simulink model "RefModel_AeroDyn_Sim"  (R2020b)
settings: Solver=ode1  StartTime=tspan(1)  StopTime=inf  FixedStep=1/sensorFs.imuUpdateFs  RelTol=1e-3  EnableMultiTasking=on
undefined symbols (not defined in the file or in its folder): ACTUATOR_SET, Earth, ENVIRONMENT_SET, F, Light, MIL, sensorFs, SIM_SENSOR_SET, UAVPARAM_SET, WGS84
libraries: simulink x10, aerolibactuator x9, aerolibnav x6, sharedutil x5, shared6dofsys x3, aerolibwind2 x2, aerolibasang x2, aerolibatmos2 x1, aerolibconvert2 x1, aerolibgravity2 x1, aerolibtransform2 x1
(part 1 of 3)
settings Model: PauseTimes=[10 20]  Creator=sl  LastModifiedBy=sl
settings SolverCC: AutoInsertRateTranBlk=on
settings OptimizationCC: DefaultParameterBehavior=Inlined  EnhancedBackFolding=on  PassReuseOutputArgsAs=Individual arguments  ZeroExternalMemoryAtStartup=off  ZeroInternalMemoryAtStartup=off  MaxStackSize=64  OptimizeBlockOrder=speed  DifferentSizesBufferReuse=on  EfficientTunableParamExpr=on
settings DebuggingCC: MultiTaskCondExecSysMsg=none  ParameterTunabilityLossMsg=error  UnconnectedInputMsg=none  UnconnectedOutputMsg=none  UnconnectedLineMsg=none
settings HardwareCC: ProdBitPerPointer=32  ProdBitPerSizeT=32  ProdBitPerPtrDiffT=32  ProdLargestAtomicInteger=Long  ProdLargestAtomicFloat=Double  ProdWordSize=32  ProdHWDeviceType=ARM Compatible->ARM Cortex
settings SFSimCC: MATLABDynamicMemAlloc=off
settings RTWCC: Description=Embedded Coder  SystemTargetFile=ert.tlc  TemplateMakefile=ert_default_tmf  GenerateReport=on  Toolchain=GNU Tools for ARM Embedded Processors  IncludeHyperlinkInReport=on  LaunchReport=on  GenerateTraceInfo=on  GenerateTraceReport=on  GenerateTraceReportSl=on  GenerateTraceReportSf=on  GenerateTraceReportEml=on
settings CodeAppCC: ForceParamTrailComments=on  IgnoreCustomStorageClasses=off  OperatorAnnotations=on  SimulinkDataObjDesc=on  SFDataObjDesc=on  InsertBlockDesc=on
settings ERTTargetCC: InlinedParameterPlacement=NonHierarchical  ERTCustomFileTemplate=example_file_process.tlc

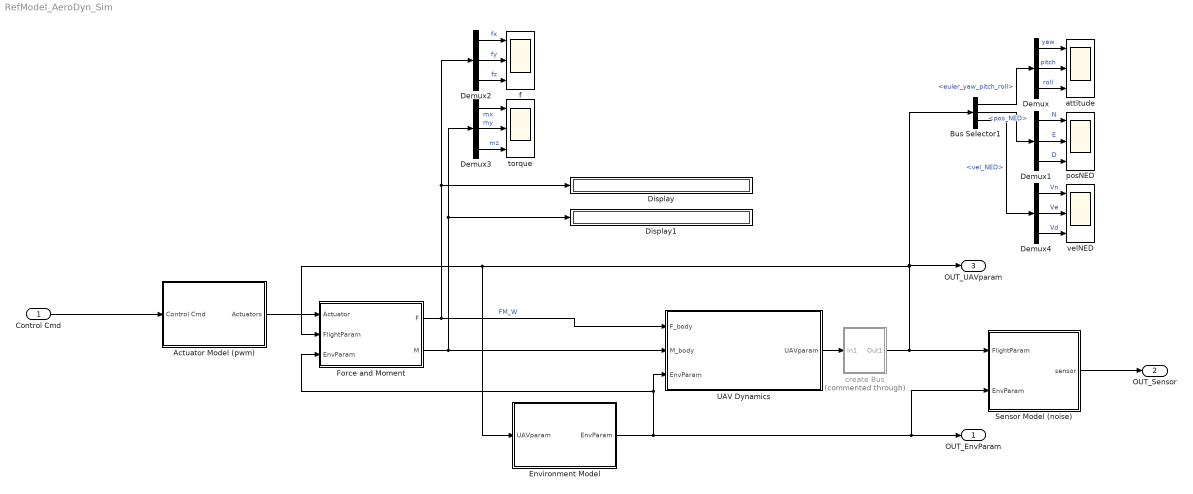
== system RefModel_AeroDyn_Sim ==
  Control Cmd : Inport  OutDataTypeStr=Bus: BUS_CONTROL_ACTUATOR  BusOutputAsStruct=on
  Actuator Model (pwm) : Subsystem
  Bus Selector1 : BusSelector  OutputSignals=euler_yaw_pitch_roll,pos_NED,vel_NED
  Demux{,1..4} (5 alike) : Demux  Outputs=3
  Display : Display
  Display1 : Display
  Environment Model : Subsystem
  Force and Moment : Subsystem
  Sensor Model (noise) : Subsystem  VariantControl=SensorNoiseMode==1
  UAV Dynamics : Subsystem
  attitude : Scope  NumInputPorts=3
  create Bus : Subsystem  Commented=through
  f : Scope  NumInputPorts=3
  posNED : Scope  NumInputPorts=3
  torque : Scope  NumInputPorts=3
  velNED : Scope  NumInputPorts=3
  OUT_EnvParam : Outport  OutDataTypeStr=Bus: BUS_UAVDYN_Env
  OUT_Sensor : Outport  Port=2  OutDataTypeStr=Bus: BUS_SENSOR
  OUT_UAVparam : Outport  Port=3  OutDataTypeStr=Bus: BUS_UAVDYN_FlightParam
  wires:
  Actuator Model (pwm)/1(Actuators) -> Force and Moment/1(Actuator)
  Environment Model/1(EnvParam) -> Force and Moment/3(EnvParam), UAV Dynamics/3(EnvParam), Sensor Model (noise)/2(EnvParam), OUT_EnvParam/1
  Control Cmd/1 -> Actuator Model (pwm)/1(Control Cmd)
  Demux/3 -> attitude/3  "roll"
  Demux/1 -> attitude/1  "yaw"
  Demux/2 -> attitude/2  "pitch"
  create Bus/1(Out1) -> OUT_UAVparam/1, Bus Selector1/1, Force and Moment/2(FlightParam), Environment Model/1(UAVparam), Sensor Model (noise)/1(FlightParam)
  Force and Moment/1(F) -> Demux2/1, Display/1, UAV Dynamics/1(F_body)  "FM_W"
  Force and Moment/2(M) -> Demux3/1, Display1/1, UAV Dynamics/2(M_body)
  Bus Selector1/2 -> Demux1/1  "<pos_NED>"
  Demux1/3 -> posNED/3  "D"
  UAV Dynamics/1(UAVparam) -> create Bus/1(In1)
  Demux1/1 -> posNED/1  "N"
  Bus Selector1/1 -> Demux/1  "<euler_yaw_pitch_roll>"
  Sensor Model (noise)/1(sensor) -> OUT_Sensor/1
  Demux1/2 -> posNED/2  "E"
  Demux3/3 -> torque/3  "mz"
  Demux2/1 -> f/1  "fx"
  Demux3/1 -> torque/1  "mx"
  Demux2/2 -> f/2  "fy"
  Demux3/2 -> torque/2  "my"
  Demux2/3 -> f/3  "fz"
  Demux4/2 -> velNED/2  "Ve"
  Demux4/1 -> velNED/1  "Vn"
  Demux4/3 -> velNED/3  "Vd"
  Bus Selector1/3 -> Demux4/1  "<vel_NED>"

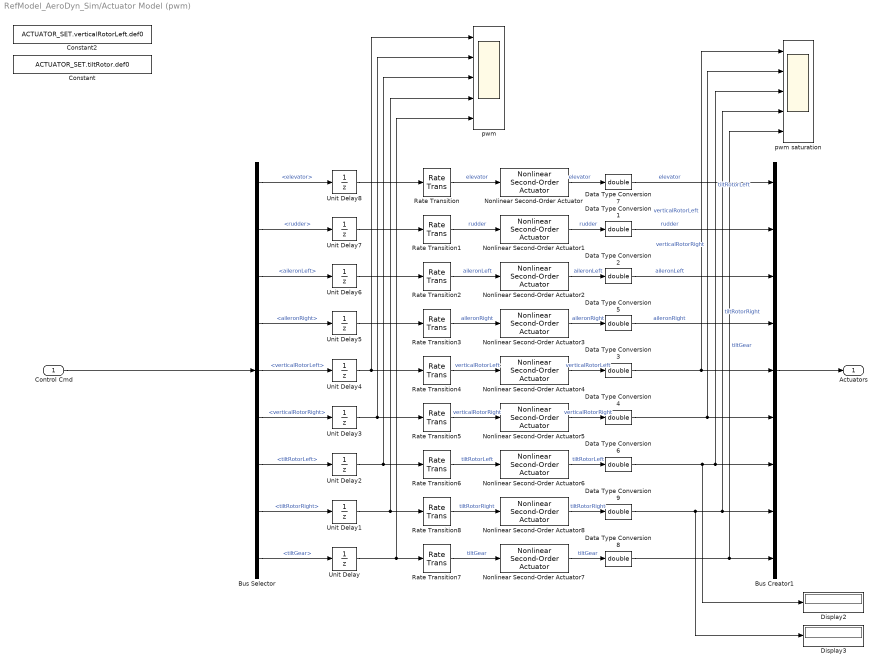
== system RefModel_AeroDyn_Sim/Actuator Model (pwm) ==
  Control Cmd : Inport
  Bus Creator1 : BusCreator  Inputs=9
  Bus Selector : BusSelector  OutputSignals=elevator,rudder,aileronLeft,aileronRight,verticalRotorLeft,verticalRotorRight,tiltRotorLeft,tiltRotorRight,tiltGear
  Constant : Constant  Value=ACTUATOR_SET.tiltRotor.def0
  Constant2 : Constant  Value=ACTUATOR_SET.verticalRotorLeft.def0
  Data Type Conversion{1..9} (9 alike) : DataTypeConversion  OutDataTypeStr=double
  Display2 : Display
  Display3 : Display
  Nonlinear Second-Order Actuator : aerolibactuator/Nonlinear Second-Order Actuator  wn_fin=ACTUATOR_SET.elevator.naturalFreq  z_fin=ACTUATOR_SET.elevator.dampingRatio  fin_max=ACTUATOR_SET.elevator.def_max  fin_min=ACTUATOR_SET.elevator.def_min  fin_maxrate=ACTUATOR_SET.elevator.rateLimit  fin_act_0=ACTUATOR_SET.elevator.initialPos  fin_act_vel=0
      settings: SourceProductBaseCode=AE
  Nonlinear Second-Order Actuator1 : aerolibactuator/Nonlinear Second-Order Actuator  wn_fin=ACTUATOR_SET.rudder.naturalFreq  z_fin=ACTUATOR_SET.rudder.dampingRatio  fin_max=ACTUATOR_SET.rudder.def_max  fin_min=ACTUATOR_SET.rudder.def_min  fin_maxrate=ACTUATOR_SET.rudder.rateLimit  fin_act_0=ACTUATOR_SET.rudder.initialPos  fin_act_vel=0
      settings: SourceProductBaseCode=AE
  Nonlinear Second-Order Actuator2 : aerolibactuator/Nonlinear Second-Order Actuator  wn_fin=ACTUATOR_SET.aileronLeft.naturalFreq  z_fin=ACTUATOR_SET.aileronLeft.dampingRatio  fin_max=ACTUATOR_SET.aileronLeft.def_max  fin_min=ACTUATOR_SET.aileronLeft.def_min  fin_maxrate=ACTUATOR_SET.aileronLeft.rateLimit  fin_act_0=ACTUATOR_SET.aileronLeft.initialPos  fin_act_vel=0
      settings: SourceProductBaseCode=AE
  Nonlinear Second-Order Actuator3 : aerolibactuator/Nonlinear Second-Order Actuator  wn_fin=ACTUATOR_SET.aileronRight.naturalFreq  z_fin=ACTUATOR_SET.aileronRight.dampingRatio  fin_max=ACTUATOR_SET.aileronRight.def_max  fin_min=ACTUATOR_SET.aileronRight.def_min  fin_maxrate=ACTUATOR_SET.aileronRight.rateLimit  fin_act_0=ACTUATOR_SET.aileronRight.initialPos  fin_act_vel=0
      settings: SourceProductBaseCode=AE
  Nonlinear Second-Order Actuator4 : aerolibactuator/Nonlinear Second-Order Actuator  wn_fin=ACTUATOR_SET.verticalRotor.naturalFreq_pwm  z_fin=ACTUATOR_SET.verticalRotor.dampingRatio_pwm  fin_max=ACTUATOR_SET.verticalRotor.def_max_pwm  fin_min=ACTUATOR_SET.verticalRotor.def_min_pwm  fin_maxrate=ACTUATOR_SET.verticalRotor.rateLimit_pwm  fin_act_0=ACTUATOR_SET.verticalRotor.def0_pwm  fin_act_vel=0
      settings: SourceProductBaseCode=AE
  Nonlinear Second-Order Actuator5 : aerolibactuator/Nonlinear Second-Order Actuator  wn_fin=ACTUATOR_SET.verticalRotor.naturalFreq_pwm  z_fin=ACTUATOR_SET.verticalRotor.dampingRatio_pwm  fin_max=ACTUATOR_SET.verticalRotor.def_max_pwm  fin_min=ACTUATOR_SET.verticalRotor.def_min_pwm  fin_maxrate=ACTUATOR_SET.verticalRotor.rateLimit_pwm  fin_act_0=ACTUATOR_SET.verticalRotor.def0_pwm  fin_act_vel=0
      settings: SourceProductBaseCode=AE
  Nonlinear Second-Order Actuator6 : aerolibactuator/Nonlinear Second-Order Actuator  wn_fin=ACTUATOR_SET.tiltRotor.naturalFreq_pwm  z_fin=ACTUATOR_SET.tiltRotor.dampingRatio_pwm  fin_max=ACTUATOR_SET.tiltRotor.def_max_pwm  fin_min=ACTUATOR_SET.tiltRotor.def_min_pwm  fin_maxrate=ACTUATOR_SET.tiltRotor.rateLimit_pwm  fin_act_0=ACTUATOR_SET.tiltRotor.def0_pwm  fin_act_vel=0
      settings: SourceProductBaseCode=AE
  Nonlinear Second-Order Actuator7 : aerolibactuator/Nonlinear Second-Order Actuator  wn_fin=ACTUATOR_SET.tiltGear.naturalFreq  z_fin=ACTUATOR_SET.tiltGear.dampingRatio  fin_max=ACTUATOR_SET.tiltGear.def_max  fin_min=ACTUATOR_SET.tiltGear.def_min  fin_maxrate=ACTUATOR_SET.tiltGear.rateLimit  fin_act_0=ACTUATOR_SET.tiltGear.initialPos  fin_act_vel=0
      settings: SourceProductBaseCode=AE
  Nonlinear Second-Order Actuator8 : aerolibactuator/Nonlinear Second-Order Actuator  wn_fin=ACTUATOR_SET.tiltRotor.naturalFreq_pwm  z_fin=ACTUATOR_SET.tiltRotor.dampingRatio_pwm  fin_max=ACTUATOR_SET.tiltRotor.def_max_pwm  fin_min=ACTUATOR_SET.tiltRotor.def_min_pwm  fin_maxrate=ACTUATOR_SET.tiltRotor.rateLimit_pwm  fin_act_0=ACTUATOR_SET.tiltRotor.def0_pwm  fin_act_vel=0
      settings: SourceProductBaseCode=AE
  Rate Transition{,1..8} (9 alike) : RateTransition  OutPortSampleTime=0
  Unit Delay{,1..8} (9 alike) : UnitDelay  SampleTime=-1  HasFrameUpgradeWarning=on
  pwm : Scope  NumInputPorts=5
  pwm saturation : Scope  NumInputPorts=5
  Actuators : Outport  VectorParamsAs1DForOutWhenUnconnected=off
  wires:
  Unit Delay5/1 -> Rate Transition3/1
  Unit Delay4/1 -> pwm/1, Rate Transition4/1
  Unit Delay7/1 -> Rate Transition1/1
  Unit Delay6/1 -> Rate Transition2/1
  Unit Delay8/1 -> Rate Transition/1
  Unit Delay2/1 -> pwm/3, Rate Transition6/1
  Unit Delay3/1 -> pwm/2, Rate Transition5/1
  Unit Delay1/1 -> pwm/4, Rate Transition8/1
  Unit Delay/1 -> pwm/5, Rate Transition7/1
  Control Cmd/1 -> Bus Selector/1
  Bus Selector/9 -> Unit Delay/1  "<tiltGear>"
  Bus Selector/8 -> Unit Delay1/1  "<tiltRotorRight>"
  Bus Selector/7 -> Unit Delay2/1  "<tiltRotorLeft>"
  Bus Selector/6 -> Unit Delay3/1  "<verticalRotorRight>"
  Bus Selector/5 -> Unit Delay4/1  "<verticalRotorLeft>"
  Bus Selector/4 -> Unit Delay5/1  "<aileronRight>"
  Bus Selector/3 -> Unit Delay6/1  "<aileronLeft>"
  Bus Selector/2 -> Unit Delay7/1  "<rudder>"
  Bus Selector/1 -> Unit Delay8/1  "<elevator>"
  Data Type Conversion2/1 -> Bus Creator1/3  "aileronLeft"
  Data Type Conversion9/1 -> Bus Creator1/8, pwm saturation/4, Display3/1  "tiltRotorRight"
  Data Type Conversion3/1 -> Bus Creator1/5, pwm saturation/1  "verticalRotorLeft"
  Bus Creator1/1 -> Actuators/1
  Data Type Conversion1/1 -> Bus Creator1/2  "rudder"
  Data Type Conversion6/1 -> Bus Creator1/7, pwm saturation/3, Display2/1  "tiltRotorLeft"
  Data Type Conversion8/1 -> pwm saturation/5, Bus Creator1/9  "tiltGear"
  Data Type Conversion5/1 -> Bus Creator1/4  "aileronRight"
  Data Type Conversion7/1 -> Bus Creator1/1  "elevator"
  Data Type Conversion4/1 -> Bus Creator1/6, pwm saturation/2  "verticalRotorRight"
  Rate Transition3/1 -> Nonlinear Second-Order Actuator3/1  "aileronRight"
  Rate Transition6/1 -> Nonlinear Second-Order Actuator6/1  "tiltRotorLeft"
  Rate Transition2/1 -> Nonlinear Second-Order Actuator2/1  "aileronLeft"
  Rate Transition/1 -> Nonlinear Second-Order Actuator/1  "elevator"
  Rate Transition7/1 -> Nonlinear Second-Order Actuator7/1  "tiltGear"
  Rate Transition1/1 -> Nonlinear Second-Order Actuator1/1  "rudder"
  Rate Transition8/1 -> Nonlinear Second-Order Actuator8/1  "tiltRotorRight"
  Rate Transition4/1 -> Nonlinear Second-Order Actuator4/1  "verticalRotorLeft"
  Rate Transition5/1 -> Nonlinear Second-Order Actuator5/1  "verticalRotorRight"
  Nonlinear Second-Order Actuator/1 -> Data Type Conversion7/1  "elevator"
  Nonlinear Second-Order Actuator1/1 -> Data Type Conversion1/1  "rudder"
  Nonlinear Second-Order Actuator2/1 -> Data Type Conversion2/1  "aileronLeft"
  Nonlinear Second-Order Actuator3/1 -> Data Type Conversion5/1  "aileronRight"
  Nonlinear Second-Order Actuator4/1 -> Data Type Conversion3/1  "verticalRotorLeft"
  Nonlinear Second-Order Actuator5/1 -> Data Type Conversion4/1  "verticalRotorRight"
  Nonlinear Second-Order Actuator8/1 -> Data Type Conversion9/1  "tiltRotorRight"
  Nonlinear Second-Order Actuator6/1 -> Data Type Conversion6/1  "tiltRotorLeft"
  Nonlinear Second-Order Actuator7/1 -> Data Type Conversion8/1  "tiltGear"

== system RefModel_AeroDyn_Sim/Environment Model ==
  UAVparam1 : Inport  PortName=UAVparam  Element=LLA
  UAVparam2 : Inport  PortName=UAVparam  Element=DCMbe
  UAVparam3 : Inport  PortName=UAVparam  Element=airspeed
  Atoms Model : Subsystem
  Gravity Model : Subsystem
  Selector : Selector  InputPortWidth=3  IndexOptions=Index vector (dialog)  Indices=3  OutputSizes=1
  Wind Model : Subsystem
  Out Bus Element : Outport  PortName=EnvParam  Element=Vw_ned
  Out Bus Element1 : Outport  PortName=EnvParam  Element=Vw_body
  Out Bus Element2 : Outport  PortName=EnvParam  Element=staticPressure
  Out Bus Element3 : Outport  PortName=EnvParam  Element=rho
  Out Bus Element4 : Outport  PortName=EnvParam  Element=temperature
  Out Bus Element5 : Outport  PortName=EnvParam  Element=gravity
  wires:
  UAVparam1/1 -> Gravity Model/1(LLA), Selector/1
  Selector/1 -> Wind Model/3(height), Atoms Model/1(height)
  UAVparam2/1 -> Wind Model/2(DCMbe)
  UAVparam3/1 -> Wind Model/1(speed)
  Atoms Model/1(temperature) -> Out Bus Element4/1
  Atoms Model/2(staticPressure) -> Out Bus Element2/1
  Atoms Model/3(rho) -> Out Bus Element3/1
  Gravity Model/1(gravity) -> Out Bus Element5/1
  Wind Model/1(Vwind_ned) -> Out Bus Element/1
  Wind Model/2(Vwind_body) -> Out Bus Element1/1

== system RefModel_AeroDyn_Sim/Force and Moment ==
  Actuator : Inport
  FlightParam : Inport  Port=2
  EnvParam : Inport  Port=3
  Add : Sum  Inputs=3
  Add1 : Sum  Inputs=3
  Aero Surface : Subsystem  Commented=on
  Demux : Demux  Outputs=3
  Demux1 : Demux  Outputs=3
  Display : Display
  Display1 : Display
  Gravity Force : Subsystem
  Mux : Mux  Inputs=3
  Mux1 : Mux  Inputs=3
  Rotor Force : Subsystem
  F : Outport  VectorParamsAs1DForOutWhenUnconnected=off
  M : Outport  Port=2  VectorParamsAs1DForOutWhenUnconnected=off
  wires:
  Aero Surface/1(Aero Force) -> Add/1
  Actuator/1 -> Rotor Force/1(Actuator), Aero Surface/1(ActuatorParam)
  FlightParam/1 -> Gravity Force/2(FlightParam), Rotor Force/2(FlightParam), Aero Surface/2(FlightParam)
  EnvParam/1 -> Gravity Force/1(EnvParam)
  Gravity Force/1(Gravity Force) -> Add/3
  Rotor Force/1(Rotor Force) -> Add/2
  Aero Surface/2(Aero Moment) -> Add1/1
  Rotor Force/2(Rotor Moment) -> Add1/2
  Gravity Force/2(Gravity Moment) -> Add1/3
  Add1/1 -> Display/1, Demux/1
  Mux/1 -> M/1
  Add/1 -> Display1/1, Demux1/1
  Mux1/1 -> F/1
  Demux/3 -> Mux/3
  Demux/2 -> Mux/2
  Demux/1 -> Mux/1
  Demux1/1 -> Mux1/1
  Demux1/2 -> Mux1/2
  Demux1/3 -> Mux1/3

== system RefModel_AeroDyn_Sim/Sensor Model (noise) ==
  FlightParam : Inport
  EnvParam : Inport  Port=2
  Airspeed1 : Subsystem
  Baro1 : Subsystem
  Bus Creator : BusCreator  Inputs=11
  Constant : Constant  Value=SIM_SENSOR_SET.NoiseEnable
  Digital Clock : DigitalClock  SampleTime=1/sensorFs.imuUpdateFs
  IMU1 : Subsystem  TreatAsAtomicUnit=on
  IMU2 : Subsystem  TreatAsAtomicUnit=on
  IMU3 : Subsystem  TreatAsAtomicUnit=on
  Mag1 : Subsystem
  Mag2 : Subsystem
  Radar1 : Subsystem
  Ublox1 : Subsystem
  um482 : Subsystem
  sensor : Outport
  wires:
  FlightParam/1 -> Baro1/2(In1), IMU3/2(In1), IMU2/2(In1), IMU1/2(In1), Ublox1/2(In1), Radar1/2(In1), Airspeed1/2(In1), um482/2(In1), Mag2/2(signal), Mag1/2(signal)
  Ublox1/1(GPSout) -> Bus Creator/7  "ublox1"
  Airspeed1/1(airspeed) -> Bus Creator/5  "airspeed1"
  Mag2/1(mag1) -> Bus Creator/3  "mag2"
  Bus Creator/1 -> sensor/1
  Digital Clock/1 -> Bus Creator/1  "time"
  um482/1(GPSout) -> Bus Creator/4  "um482"
  Baro1/1(altBaro1) -> Bus Creator/11  "baro1"
  Mag1/1(mag1) -> Bus Creator/2  "mag1"
  Radar1/1(range) -> Bus Creator/6  "radar1"
  IMU2/1(IMU) -> Bus Creator/9  "IMU2"
  IMU3/1(IMU) -> Bus Creator/10  "IMU3"
  IMU1/1(IMU) -> Bus Creator/8  "IMU1"
  Constant/1 -> Mag1/1(flag), Baro1/1(flag), IMU3/1(flag), IMU2/1(flag), IMU1/1(flag), Ublox1/1(flag), Radar1/1(flag), Airspeed1/1(flag), um482/1(flag), Mag2/1(flag)
  EnvParam/1 -> Mag1/3(In3), Airspeed1/3(In3), Baro1/3(In3), IMU3/3(In3), IMU2/3(In3), IMU1/3(In3), Ublox1/3(In3), Radar1/3(In3), um482/3(In3), Mag2/3(In3)

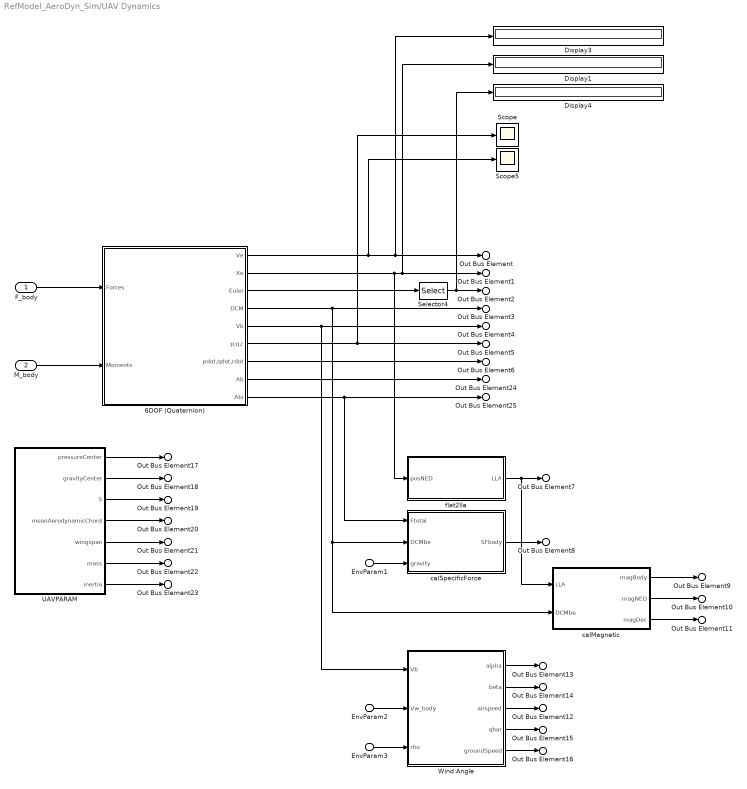
== system RefModel_AeroDyn_Sim/UAV Dynamics ==
  F_body : Inport
  M_body : Inport  Port=2
  EnvParam1 : Inport  Port=3  PortName=EnvParam  Element=gravity
  EnvParam2 : Inport  Port=3  PortName=EnvParam  Element=Vw_body
  EnvParam3 : Inport  Port=3  PortName=EnvParam  Element=rho
  6DOF (Quaternion) : Subsystem  AncestorBlock=shared6dof/6DOF (Euler Angles)  mask(6DOF EoM (Body Axis)){units=Metric (MKS), mtype=Fixed, rep=Quaternion, xme_0=[0,0,0], Vm_0=UAVPARAM_SET.gpsvel0, eul_0=UAVPARAM_SET.euler0_roll_pitch_yaw, pm_0=[0,0,0], mass_0=UAVPARAM_SET.mass, mass_e=0.5, mass_f=2.0, inertia=UAVPARAM_SET.inertia, inertia_e=eye(3), inertia_f=2*eye(3), k_quat=1.0, vre_flag=on, abi_flag=on, aMode=0, xme_statename='', Vm_statename='', eul_statename='', quat_statename='', pm_statename='', mass_statename=''}
      mask prompts: units "shared_aeroblks:sharedaeroblk6dofbody:block6DOFEoMBodyAxisParamUnits"; mtype "shared_aeroblks:sharedaeroblk6dofbody:block6DOFEoMBodyAxisParamMasstype"; rep "shared_aeroblks:sharedaeroblk6dofbody:block6DOFEoMBodyAxisParamRepresentation"; xme_0 "shared_aeroblks:sharedaeroblk6dofbody:block6DOFEoMBodyAxisParamInitialpositionininertialaxesXeYeZe"; Vm_0 "shared_aeroblks:sharedaeroblk6dofbody:block6DOFEoMBodyAxisParamInitialvelocityinbodyaxesUvw"; eul_0 "shared_aeroblks:sharedaeroblk6dofbody:block6DOFEoMBodyAxisParamInitialEulerorientationrollpitchyaw"; pm_0 "shared_aeroblks:sharedaeroblk6dofbody:block6DOFEoMBodyAxisParamInitialbodyrotationratespqr"; mass_0 "shared_aeroblks:sharedaeroblk6dofbody:block6DOFEoMBodyAxisParamInitialmass"; mass_e "shared_aeroblks:sharedaeroblk6dofbody:block6DOFEoMBodyAxisParamEmptymass"; mass_f "shared_aeroblks:sharedaeroblk6dofbody:block6DOFEoMBodyAxisParamFullmass"; inertia "shared_aeroblks:sharedaeroblk6dofbody:block6DOFEoMBodyAxisParamInertia"; inertia_e "shared_aeroblks:sharedaeroblk6dofbody:block6DOFEoMBodyAxisParamEmptyinertiamatrix"; inertia_f "shared_aeroblks:sharedaeroblk6dofbody:block6DOFEoMBodyAxisParamFullinertiamatrix"; k_quat "shared_aeroblks:sharedaeroblk6dofbody:block6DOFEoMBodyAxisParamGainforquaternionnormalization"; vre_flag "shared_aeroblks:sharedaeroblk6dofbody:block6DOFEoMBodyAxisParamIncludemassflowrelativevelocity"; abi_flag "shared_aeroblks:sharedaeroblk6dofbody:inertialAccelFlag"; xme_statename "shared_aeroblks:sharedaeroblk6dofbody:block6DOFEoMStateNamePosition"; Vm_statename "shared_aeroblks:sharedaeroblk6dofbody:block6DOFEoMStateNameVelocity"; eul_statename "shared_aeroblks:sharedaeroblk6dofbody:block6DOFEoMStateNameEulerAngles"; quat_statename "shared_aeroblks:sharedaeroblk6dofbody:block6DOFEoMStateNameQuaternions"; pm_statename "shared_aeroblks:sharedaeroblk6dofbody:block6DOFEoMStateNameRotationRates"; mass_statename "shared_aeroblks:sharedaeroblk6dofbody:block6DOFEoMStateNameMass"
      mask help: shared_aeroblks:sharedaeroblk6dofbody:block6DOFEoMBodyAxisDesc
      mask init:
      | if aerosharedtest(gcb)
      |     ports=aerosharedicon('shared6dofbody','icon');
      | else
      |     ports=sharedautoicon('shared6dofbody','icon');
      | end
      mask Help: eval('aerosharedhelp(''sixdof_quaternion'')');
      mask TypeOptions units: shared_aeroblks:sharedaeroblk6dofbody:block6DOFEoMBodyAxisParamComboMetricMKS | shared_aeroblks:sharedaeroblk6dofbody:block6DOFEoMBodyAxisParamComboEnglishVelocityinfts | shared_aeroblks:sharedaeroblk6dofbody:block6DOFEoMBodyAxisParamComboEnglishVelocityinkts
      mask TypeOptions mtype: shared_aeroblks:sharedaeroblk6dofbody:block6DOFEoMBodyAxisParamComboFixed | shared_aeroblks:sharedaeroblk6dofbody:block6DOFEoMBodyAxisParamComboSimpleVariable | shared_aeroblks:sharedaeroblk6dofbody:block6DOFEoMBodyAxisParamComboCustomVariable
      mask Callback mtype:
      | if aerosharedtest(gcb) && builtin('license','test','aerospace_blockset')
      |     aerosharedicon('shared6dofbody');
      | else
      |     sharedautoicon('shared6dofbody');
      | end
      mask TypeOptions rep: shared_aeroblks:sharedaeroblk6dofbody:block6DOFEoMBodyAxisParamComboEulerAngles | shared_aeroblks:sharedaeroblk6dofbody:block6DOFEoMBodyAxisParamComboQuaternion
      mask Callback rep:
      | if aerosharedtest(gcb) && builtin('license','test','aerospace_blockset')
      |     aerosharedicon('shared6dofbody');
      | else
      |     sharedautoicon('shared6dofbody');
      | end
      mask DialogControl Container4 Prompt: shared_aeroblks:sharedaeroblk6dofbody:block6DOFEoMParamTab
      mask DialogControl units Prompt: Units:
      mask DialogControl mtype Prompt: Mass type:
      mask DialogControl rep Prompt: Representation:
      mask DialogControl xme_0 Prompt: Initial position in inertial axes [Xe,Ye,Ze]:
      mask DialogControl Vm_0 Prompt: Initial velocity in body axes [U,v,w]:
      mask DialogControl eul_0 Prompt: Initial Euler orientation [roll, pitch, yaw]:
      mask DialogControl pm_0 Prompt: Initial body rotation rates [p,q,r]:
      mask DialogControl mass_0 Prompt: Initial mass:
      mask DialogControl mass_e Prompt: Empty mass:
      mask DialogControl mass_f Prompt: Full mass:
      mask DialogControl inertia Prompt: Inertia:
      mask DialogControl inertia_e Prompt: Empty inertia matrix:
      mask DialogControl inertia_f Prompt: Full inertia matrix:
      mask DialogControl k_quat Prompt: Gain for quaternion normalization:
      mask DialogControl vre_flag Prompt: Include mass flow relative velocity
      mask DialogControl abi_flag Prompt: Include inertial acceleration
      mask DialogControl Container6 Prompt: shared_aeroblks:sharedaeroblk6dofbody:block6DOFEoMStateAttributesTab
      mask DialogControl Container7 Prompt: shared_aeroblks:sharedaeroblk6dofbody:block6DOFEoMStateNamesGroup
      mask DialogControl xme_statename Prompt: Position: e.g., {'Xe', 'Ye', 'Ze'}
      mask DialogControl Vm_statename Prompt: Velocity: e.g., {'U', 'v', 'w'}
      mask DialogControl eul_statename Prompt: Euler rotation angles: e.g., {'phi', 'theta', 'psi'}
      mask DialogControl quat_statename Prompt: Quaternion vector: e.g., {'qr', 'qi', 'qj', 'qk'}
      mask DialogControl pm_statename Prompt: Body rotation rates: e.g., {'p', 'q', 'r'}
      mask DialogControl mass_statename Prompt: Mass: e.g., 'mass'
      mask Display:
      | port_label(ports(1).type,ports(1).port,ports(1).txt,'texmode','on');
      | port_label(ports(2).type,ports(2).port,ports(2).txt,'texmode','on');
      | port_label(ports(3).type,ports(3).port,ports(3).txt,'texmode','on');
      | port_label(ports(4).type,ports(4).port,ports(4).txt,'texmode','on');
      | port_label(ports(5).type,ports(5).port,ports(5).txt,'texmode','on');
      | port_label(ports(6).type,ports(6).port,ports(6).txt,'texmode','on');
      | port_label(ports(7).type,ports(7).port,ports(7).txt,'texmode','on');
      | port_label(ports(8).type,ports(8).port,ports(8).txt,'texmode','on');
      | port_label(ports(9).type,ports(9).port,ports(9).txt,'texmode','on');
      | port_label(ports(10).type,ports(10).port,ports(10).txt,'texmode','on');
      | port_label(ports(11).type,ports(11).port,ports(11).txt,'texmode','on');
      | port_label(ports(12).type,ports(12).port,ports(12).txt,'texmode','on');
      | port_label(ports(13).type,ports(13).port,ports(13).txt,'texmode','on');
      | port_label(ports(14).type,ports(14).port,ports(14).txt,'texmode','on');
      | port_label(ports(15).type,ports(15).port,ports(15).txt,'texmode','on');
      | port_label(ports(16).type,ports(16).port,ports(16).txt,'texmode','on');
      | port_label(ports(17).type,ports(17).port,ports(17).txt,'texmode','on');
  Display1 : Display
  Display3 : Display
  Display4 : Display
  Scope : Scope
  Scope5 : Scope
  Selector4 : Selector  InputPortWidth=3  IndexOptions=Index vector (dialog)  Indices=[3 2 1]  OutputSizes=1
  UAVPARAM : Subsystem
  Wind Angle : Subsystem  TreatAsAtomicUnit=on  VariantControl=use_aerospace_blocks == 1
  calMagnetic : Subsystem
  calSpecificForce : Subsystem
  flat2lla : Subsystem
  Out Bus Element : Outport  PortName=UAVparam  Element=vel_NED
  Out Bus Element1 : Outport  PortName=UAVparam  Element=pos_NED
  Out Bus Element2 : Outport  PortName=UAVparam  Element=euler_yaw_pitch_roll
  Out Bus Element3 : Outport  PortName=UAVparam  Element=DCMbe
  Out Bus Element4 : Outport  PortName=UAVparam  Element=vel_Body
  Out Bus Element5 : Outport  PortName=UAVparam  Element=w_Body
  Out Bus Element6 : Outport  PortName=UAVparam  Element=dw_Body
  Out Bus Element24 : Outport  PortName=UAVparam  Element=acc_Body
  Out Bus Element25 : Outport  PortName=UAVparam  Element=acc_NED
  Out Bus Element7 : Outport  PortName=UAVparam  Element=LLA
  Out Bus Element8 : Outport  PortName=UAVparam  Element=specificForce_Body
  Out Bus Element9 : Outport  PortName=UAVparam  Element=mag_Body
  Out Bus Element10 : Outport  PortName=UAVparam  Element=mag_NED
  Out Bus Element11 : Outport  PortName=UAVparam  Element=magDec_deg
  Out Bus Element12 : Outport  PortName=UAVparam  Element=airspeed
  Out Bus Element13 : Outport  PortName=UAVparam  Element=alpha
  Out Bus Element14 : Outport  PortName=UAVparam  Element=beta
  Out Bus Element15 : Outport  PortName=UAVparam  Element=qbar
  Out Bus Element16 : Outport  PortName=UAVparam  Element=groundSpeed
  Out Bus Element17 : Outport  PortName=UAVparam  Element=pressureCenter
  Out Bus Element18 : Outport  PortName=UAVparam  Element=gravityCenter
  Out Bus Element19 : Outport  PortName=UAVparam  Element=S
  Out Bus Element20 : Outport  PortName=UAVparam  Element=meanAerodynamicChord
  Out Bus Element21 : Outport  PortName=UAVparam  Element=wingspan
  Out Bus Element22 : Outport  PortName=UAVparam  Element=mass
  Out Bus Element23 : Outport  PortName=UAVparam  Element=inertia
  wires:
  6DOF (Quaternion)/3(Euler) -> Selector4/1
  6DOF (Quaternion)/4(DCM) -> Out Bus Element3/1, calMagnetic/2(DCMbe), calSpecificForce/2(DCMbe)
  6DOF (Quaternion)/2(Xe) -> Out Bus Element1/1, Display1/1, flat2lla/1(posNED)
  6DOF (Quaternion)/6(p,q,r) -> Scope/1, Out Bus Element5/1
  calSpecificForce/1(SFbody) -> Out Bus Element8/1
  Selector4/1 -> Out Bus Element2/1, Display4/1
  6DOF (Quaternion)/7(pdot,qdot,rdot) -> Out Bus Element6/1
  calMagnetic/1(magBody) -> Out Bus Element9/1
  calMagnetic/2(magNED) -> Out Bus Element10/1
  M_body/1 -> 6DOF (Quaternion)/2(Moments)
  calMagnetic/3(magDec) -> Out Bus Element11/1
  F_body/1 -> 6DOF (Quaternion)/1(Forces)
  6DOF (Quaternion)/5(Vb) -> Wind Angle/1(Vb), Out Bus Element4/1
  flat2lla/1(LLA) -> Out Bus Element7/1, calMagnetic/1(LLA)
  6DOF (Quaternion)/9(Abi) -> Out Bus Element25/1, calSpecificForce/1(Ftotal)
  6DOF (Quaternion)/1(Ve) -> Scope5/1, Out Bus Element/1, Display3/1
  Wind Angle/1(alpha) -> Out Bus Element13/1
  Wind Angle/3(airspeed) -> Out Bus Element12/1
  Wind Angle/2(beta) -> Out Bus Element14/1
  6DOF (Quaternion)/8(Ab) -> Out Bus Element24/1
  EnvParam1/1 -> calSpecificForce/3(gravity)
  EnvParam2/1 -> Wind Angle/2(Vw_body)
  EnvParam3/1 -> Wind Angle/3(rho)
  Wind Angle/4(qbar) -> Out Bus Element15/1
  Wind Angle/5(groundSpeed) -> Out Bus Element16/1
  UAVPARAM/1(pressureCenter) -> Out Bus Element17/1
  UAVPARAM/2(gravityCenter) -> Out Bus Element18/1
  UAVPARAM/3(S) -> Out Bus Element19/1
  UAVPARAM/4(meanAerodynamicChord) -> Out Bus Element20/1
  UAVPARAM/5(wingspan) -> Out Bus Element21/1
  UAVPARAM/6(mass) -> Out Bus Element22/1
  UAVPARAM/7(inertia) -> Out Bus Element23/1

== system RefModel_AeroDyn_Sim/create Bus ==
  In1 : Inport
  Bus Creator : BusCreator  Inputs=24
  Bus Selector : BusSelector  OutputSignals=vel_NED,pos_NED,euler_yaw_pitch_roll,DCMbe,vel_Body,w_Body,dw_Body,LLA,specificForce_Body,mag_Body,mag_NED,magDec_deg,airspeed,alpha,beta,qbar,groundSpeed,pressureCenter,gravityCenter,S,meanAerodynamicChord,wingspan,mass,inertia
  Out1 : Outport
  wires:
  In1/1 -> Bus Selector/1
  Bus Selector/1 -> Bus Creator/1  "<vel_NED>"
  Bus Selector/2 -> Bus Creator/2  "<pos_NED>"
  Bus Selector/3 -> Bus Creator/3  "<euler_yaw_pitch_roll>"
  Bus Selector/4 -> Bus Creator/4  "<DCMbe>"
  Bus Selector/5 -> Bus Creator/5  "<vel_Body>"
  Bus Selector/6 -> Bus Creator/6  "<w_Body>"
  Bus Selector/7 -> Bus Creator/7  "<dw_Body>"
  Bus Selector/8 -> Bus Creator/8  "<LLA>"
  Bus Selector/9 -> Bus Creator/9  "<specificForce_Body>"
  Bus Selector/10 -> Bus Creator/10  "<mag_Body>"
  Bus Selector/11 -> Bus Creator/11  "<mag_NED>"
  Bus Selector/12 -> Bus Creator/12  "<magDec_deg>"
  Bus Selector/13 -> Bus Creator/13  "<airspeed>"
  Bus Selector/14 -> Bus Creator/14  "<alpha>"
  Bus Selector/15 -> Bus Creator/15  "<beta>"
  Bus Selector/16 -> Bus Creator/16  "<qbar>"
  Bus Selector/17 -> Bus Creator/17  "<groundSpeed>"
  Bus Selector/18 -> Bus Creator/18  "<pressureCenter>"
  Bus Selector/19 -> Bus Creator/19  "<gravityCenter>"
  Bus Selector/20 -> Bus Creator/20  "<S>"
  Bus Selector/21 -> Bus Creator/21  "<meanAerodynamicChord>"
  Bus Selector/22 -> Bus Creator/22  "<wingspan>"
  Bus Creator/1 -> Out1/1
  Bus Selector/23 -> Bus Creator/23  "<mass>"
  Bus Selector/24 -> Bus Creator/24  "<inertia>"

== system RefModel_AeroDyn_Sim/Environment Model/Atoms Model ==
  height : Inport
  ISA Atmosphere Model1 : aerolibatmos2/ISA Atmosphere Model  custom=off  g=9.80665  gamma=1.4  R=287.0531  L=0.0065  h_trop=11000  h_strat=20000  rho0=1.225  P0=101325  T0=288.15  h0=0
  Temperature Conversion : aerolibconvert2/Temperature Conversion  IU=K  OU=C
      settings: SourceProductBaseCode=AE
  Terminator1 : Terminator
  temperature : Outport
  staticPressure : Outport  Port=2
  rho : Outport  Port=3
  wires:
  Temperature Conversion/1 -> temperature/1
  ISA Atmosphere Model1/1 -> Temperature Conversion/1  "OAT"
  ISA Atmosphere Model1/2 -> Terminator1/1
  ISA Atmosphere Model1/3 -> staticPressure/1  "static"
  ISA Atmosphere Model1/4 -> rho/1
  height/1 -> ISA Atmosphere Model1/1

== system RefModel_AeroDyn_Sim/Environment Model/Gravity Model ==
  LLA : Inport
  Constant : Constant  Value=ENVIRONMENT_SET.gravity
  Terminator : Terminator
  gravity : Outport
  wires:
  LLA/1 -> Terminator/1
  Constant/1 -> gravity/1

== system RefModel_AeroDyn_Sim/Environment Model/Wind Model ==
  speed : Inport
  DCMbe : Inport  Port=2
  height : Inport  Port=3
  Add : Sum  Inputs=2
  Constant : Constant  Value=ENVIRONMENT_SET.windVel
  Constant1 : Constant  Value=ENVIRONMENT_SET.windAngle
  Dryden Wind Turbulence Model (Discrete (+q -r)) : aerolibwind2/Dryden Wind Turbulence Model  (Continuous (+q -r))  units=Metric (MKS)  spec=MIL-F-8785C  model=Discrete Dryden (+q -r)  W20=10  Wdeg=0  TurbProb=10^-2 - Light  L_high=533.4  Wingspan=1/100  ts=1/sensorFs.imuUpdateFs  Seed=[23341 23342 23343 23344]  T_on=on
  Horizontal Wind Model : aerolibwind2/Horizontal Wind Model  units=Metric (MKS)  Vw_source=External  Vwind=5  W_source=External  Wdeg=0
      settings: SourceProductBaseCode=AE
  Reduce Z Wind : Gain  Gain=[1 1 0.1]
      settings: AttributesFormatString=%<Gain>
  Rotate to E Frame : Product  Multiplication=Matrix(*)
  Subsystem : Subsystem
  Subsystem1 : Subsystem
  Terminator : Terminator
  Transpose : Math  Operator=transpose  SignedPower=on  SaturateOnIntegerOverflow=on
  Vwind_ned : Outport
  Vwind_body : Outport  Port=2
  wires:
  DCMbe/1 -> Horizontal Wind Model/1, Transpose/1, Dryden Wind Turbulence Model (Discrete (+q -r))/3
  Reduce Z Wind/1 -> Add/1
  Dryden Wind Turbulence Model (Discrete (+q -r))/1 -> Reduce Z Wind/1
  Horizontal Wind Model/1 -> Add/2
  Dryden Wind Turbulence Model (Discrete (+q -r))/2 -> Terminator/1
  Transpose/1 -> Rotate to E Frame/1
  Add/1 -> Subsystem1/1(In1), Rotate to E Frame/2
  Constant/1 -> Horizontal Wind Model/2
  Constant1/1 -> Horizontal Wind Model/3
  height/1 -> Dryden Wind Turbulence Model (Discrete (+q -r))/1
  speed/1 -> Dryden Wind Turbulence Model (Discrete (+q -r))/2
  Rotate to E Frame/1 -> Subsystem/1(In1)
  Subsystem/1(Out1) -> Vwind_ned/1
  Subsystem1/1(Out1) -> Vwind_body/1

== system RefModel_AeroDyn_Sim/Force and Moment/Aero Surface ==
  In Bus Element5 : Inport  PortName=ActuatorParam  Element=aileronLeft
  In Bus Element4 : Inport  PortName=ActuatorParam  Element=aileronRight
  In Bus Element6 : Inport  PortName=ActuatorParam  Element=rudder
  In Bus Element11 : Inport  PortName=ActuatorParam  Element=elevator
  In Bus Element1 : Inport  Port=2  PortName=FlightParam  Element=beta
  In Bus Element : Inport  Port=2  PortName=FlightParam  Element=alpha
  In Bus Element2 : Inport  Port=2  PortName=FlightParam  Element=airspeed
  In Bus Element3 : Inport  Port=2  PortName=FlightParam  Element=w_Body
  In Bus Element12 : Inport  Port=2  PortName=FlightParam  Element=qbar
  In Bus Element13 : Inport  Port=2  PortName=FlightParam  Element=S
  In Bus Element14 : Inport  Port=2  PortName=FlightParam  Element=meanAerodynamicChord
  In Bus Element15 : Inport  Port=2  PortName=FlightParam  Element=wingspan
  Bus Creator1 : BusCreator  Inputs=2
  Get Forces and Moments : Subsystem
  Lateral Channel : Subsystem
  Longitudinal Channel : Subsystem
  Aero Force : Outport
  Aero Moment : Outport  Port=2
  wires:
  In Bus Element11/1 -> Longitudinal Channel/4(elevator)
  Bus Creator1/1 -> Get Forces and Moments/5(AeroCoeffs)
  In Bus Element15/1 -> Lateral Channel/8(wingspan), Get Forces and Moments/4(wingspan)
  In Bus Element1/1 -> Longitudinal Channel/1(beta), Lateral Channel/1(beta)
  In Bus Element2/1 -> Longitudinal Channel/3(airpseed), Lateral Channel/3(airspeed)
  In Bus Element3/1 -> Longitudinal Channel/5(p,q,r), Lateral Channel/7(p,q,r)
  In Bus Element14/1 -> Longitudinal Channel/6(meanAerodynamicChord), Get Forces and Moments/3(meanAerodynamicChord)
  In Bus Element13/1 -> Get Forces and Moments/2(S)
  Get Forces and Moments/1(F_aero) -> Aero Force/1
  In Bus Element/1 -> Longitudinal Channel/2(alpha), Lateral Channel/2(alpha)
  In Bus Element5/1 -> Lateral Channel/4(aileronLeft)
  Lateral Channel/1(Lateral) -> Bus Creator1/1
  Longitudinal Channel/1(Longitudinal) -> Bus Creator1/2
  In Bus Element6/1 -> Lateral Channel/6(rudder)
  In Bus Element12/1 -> Get Forces and Moments/1(q)
  In Bus Element4/1 -> Lateral Channel/5(aileronRight)
  Get Forces and Moments/2(M_aero) -> Aero Moment/1

== system RefModel_AeroDyn_Sim/Force and Moment/Gravity Force ==
  EnvParam : Inport
  FlightParam : Inport  Port=2
  Bus Selector1 : BusSelector  OutputSignals=DCMbe,mass
  Bus Selector2 : BusSelector  OutputSignals=gravity
  Constant1 : Constant  Value=[0;0;0]
  Display : Display
  Display2 : Display
  Display3 : Display
  Divide : Product  Inputs=**  Multiplication=Matrix(*)
  Divide1 : Product  Inputs=**
  Gravity Force : Outport
  Gravity Moment : Outport  Port=2
  wires:
  EnvParam/1 -> Bus Selector2/1
  FlightParam/1 -> Bus Selector1/1
  Bus Selector1/1 -> Divide/1  "<DCMbe>"
  Divide/1 -> Display2/1, Gravity Force/1
  Constant1/1 -> Gravity Moment/1
  Divide1/1 -> Display3/1, Divide/2
  Bus Selector1/2 -> Divide1/1  "<mass>"
  Bus Selector2/1 -> Display/1, Divide1/2  "<gravity>"

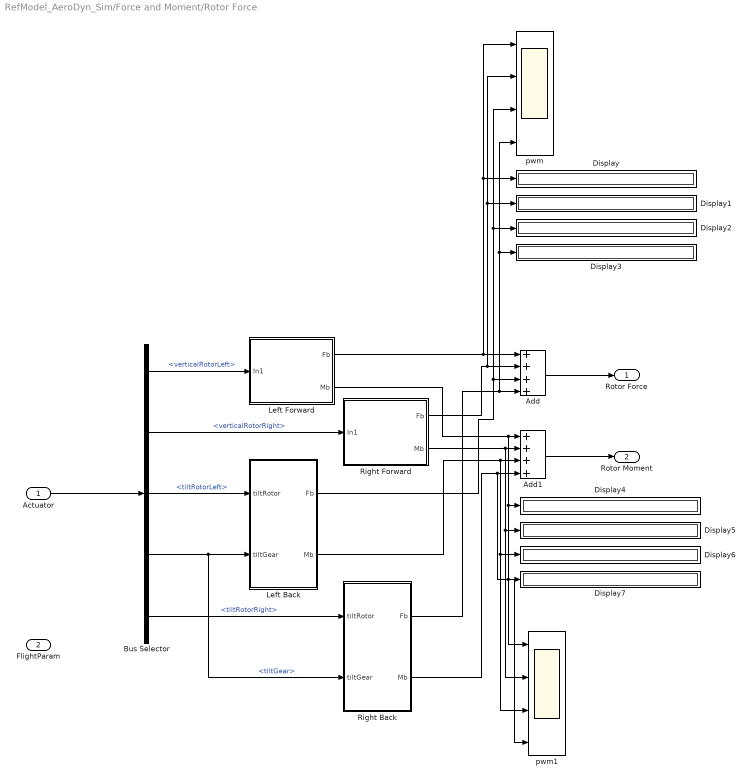
== system RefModel_AeroDyn_Sim/Force and Moment/Rotor Force ==
  Actuator : Inport
  FlightParam : Inport  Port=2
  Add : Sum  Inputs=4
  Add1 : Sum  Inputs=4
  Bus Selector : BusSelector  OutputSignals=verticalRotorLeft,verticalRotorRight,tiltRotorLeft,tiltGear,tiltRotorRight
  Display{,1..7} (8 alike) : Display
  Left Back : Subsystem
  Left Forward : Subsystem
  Right Back : Subsystem
  Right Forward : Subsystem
  pwm : Scope  NumInputPorts=4
  pwm1 : Scope  NumInputPorts=4
  Rotor Force : Outport
  Rotor Moment : Outport  Port=2
  wires:
  Add/1 -> Rotor Force/1
  Actuator/1 -> Bus Selector/1
  Bus Selector/1 -> Left Forward/1(In1)  "<verticalRotorLeft>"
  Bus Selector/2 -> Right Forward/1(In1)  "<verticalRotorRight>"
  Bus Selector/3 -> Left Back/1(tiltRotor)  "<tiltRotorLeft>"
  Left Forward/1(Fb) -> pwm/1, Display/1, Add/1
  Right Forward/1(Fb) -> pwm/2, Display1/1, Add/2
  Left Back/1(Fb) -> pwm/3, Display2/1, Add/3
  Right Forward/2(Mb) -> pwm1/2, Display5/1, Add1/2
  Left Forward/2(Mb) -> pwm1/1, Display4/1, Add1/1
  Left Back/2(Mb) -> pwm1/3, Display6/1, Add1/3
  Add1/1 -> Rotor Moment/1
  Bus Selector/4 -> Right Back/2(tiltGear), Left Back/2(tiltGear)  "<tiltGear>"
  Bus Selector/5 -> Right Back/1(tiltRotor)  "<tiltRotorRight>"
  Right Back/1(Fb) -> pwm/4, Display3/1, Add/4
  Right Back/2(Mb) -> pwm1/4, Display7/1, Add1/4

== system RefModel_AeroDyn_Sim/Sensor Model (noise)/Airspeed1 ==
  flag : Inport
  In1 : Inport  Port=2
  In3 : Inport  Port=3
  Add : Sum  Inputs=+-
  Bus Selector : BusSelector  OutputSignals=pos_NED
  Gain : Gain  Gain=-1
  Scope8 : Scope  NumInputPorts=2
  Selector : Selector  InputPortWidth=3  IndexOptions=Index vector (dialog)  Indices=3  OutputSizes=1
  Subsystem : Subsystem
  Subsystem3 : Subsystem  mask{sample_freq=sensorFs.radarUpdateFs}
      mask prompts: sample_freq "采样频率(Hz)"
  add noise1 : Subsystem
  signalBus : Subsystem
  airspeed : Outport
  wires:
  signalBus/1(airspeed1) -> airspeed/1
  Subsystem3/1(zeroHold) -> signalBus/2(airspeed)
  Add/1 -> Scope8/2
  Subsystem/1(Outport) -> Scope8/1
  Gain/1 -> add noise1/2(signal), Add/1, Subsystem/1(Inport)
  add noise1/1(Out1) -> Subsystem3/1(In), Add/2, Subsystem/2(Inport1)
  In1/1 -> Bus Selector/1
  Bus Selector/1 -> Selector/1  "<pos_NED>"
  Selector/1 -> Gain/1
  flag/1 -> add noise1/1(noise_flag)

== system RefModel_AeroDyn_Sim/Sensor Model (noise)/Baro1 ==
  flag : Inport
  In1 : Inport  Port=2
  In3 : Inport  Port=3
  Add : Sum  Inputs=+-
  Bus Selector : BusSelector  OutputSignals=pos_NED
  Gain : Gain  Gain=-1
  Scope8 : Scope  NumInputPorts=2
  Selector : Selector  InputPortWidth=3  IndexOptions=Index vector (dialog)  Indices=3  OutputSizes=1
  Subsystem : Subsystem
  Subsystem3 : Subsystem  mask{sample_freq=sensorFs.baroUpdateFs}
      mask prompts: sample_freq "采样频率(Hz)"
  add noise : Subsystem
  signalBus : Subsystem
  altBaro1 : Outport
  wires:
  In1/1 -> Bus Selector/1
  Bus Selector/1 -> Selector/1  "<pos_NED>"
  Selector/1 -> Gain/1
  Gain/1 -> Subsystem/1(Inport), Add/1, add noise/2(signal)
  add noise/1(Out1) -> Subsystem3/1(In), Subsystem/2(Inport1), Add/2
  Subsystem/1(Outport) -> Scope8/1
  Add/1 -> Scope8/2
  Subsystem3/1(zeroHold) -> signalBus/2(alt_baro)
  ? -> signalBus/1(time)
  signalBus/1(baro1) -> altBaro1/1  "baro1"
  flag/1 -> add noise/1(noise_flag)

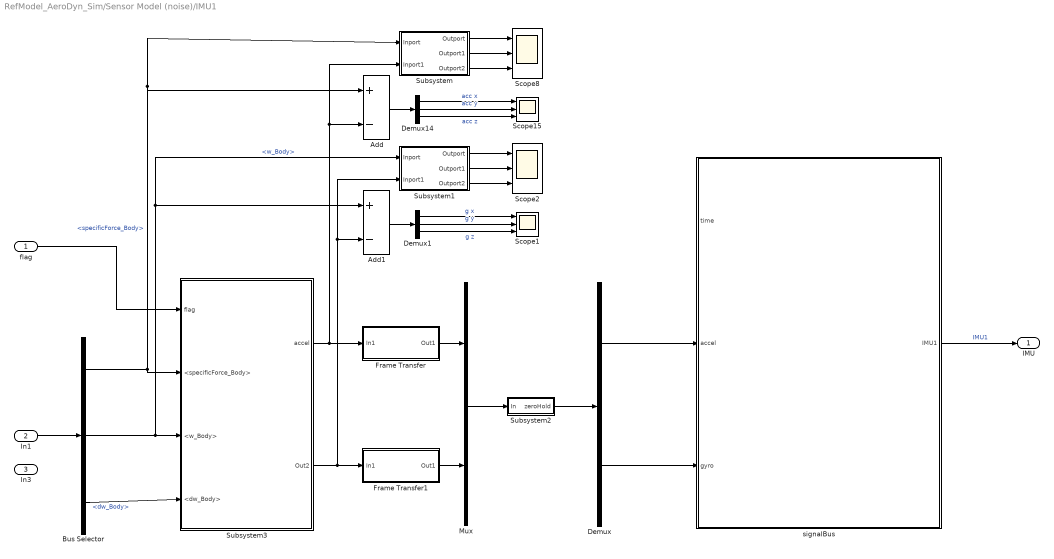
== system RefModel_AeroDyn_Sim/Sensor Model (noise)/IMU1 ==
  flag : Inport
  In1 : Inport  Port=2
  In3 : Inport  Port=3
  Add : Sum  Inputs=+-
  Add1 : Sum  Inputs=+-
  Bus Selector : BusSelector  OutputSignals=specificForce_Body,w_Body,dw_Body
  Demux : Demux  Outputs=2
  Demux1 : Demux  Outputs=3
  Demux14 : Demux  Outputs=3
  Frame Transfer : Subsystem
  Frame Transfer1 : Subsystem
  Mux : Mux  Inputs=2
  Scope{1..2,8,15} (4 alike) : Scope  NumInputPorts=3
  Subsystem : Subsystem
  Subsystem1 : Subsystem
  Subsystem2 : Subsystem  mask{sample_freq=sensorFs.imuUpdateFs}
      mask prompts: sample_freq "采样频率(Hz)"
  Subsystem3 : Subsystem
  signalBus : Subsystem
  IMU : Outport
  wires:
  In1/1 -> Bus Selector/1
  Bus Selector/2 -> Add1/1, Subsystem1/1(Inport), Subsystem3/3(<w_Body>)  "<w_Body>"
  Bus Selector/1 -> Add/1, Subsystem/1(Inport), Subsystem3/2(<specificForce_Body>)  "<specificForce_Body>"
  Add/1 -> Demux14/1
  Demux14/3 -> Scope15/3  "acc z"
  Subsystem/3(Outport2) -> Scope8/3
  Demux14/2 -> Scope15/2  "acc y"
  Demux14/1 -> Scope15/1  "acc x"
  Subsystem/1(Outport) -> Scope8/1
  Subsystem/2(Outport1) -> Scope8/2
  Subsystem1/2(Outport1) -> Scope2/2
  Subsystem1/1(Outport) -> Scope2/1
  Demux1/1 -> Scope1/1  "g x"
  Demux1/2 -> Scope1/2  "g y"
  Subsystem1/3(Outport2) -> Scope2/3
  Demux1/3 -> Scope1/3  "g z"
  Add1/1 -> Demux1/1
  signalBus/1(IMU1) -> IMU/1  "IMU1"
  Mux/1 -> Subsystem2/1(In)
  Subsystem2/1(zeroHold) -> Demux/1
  Demux/1 -> signalBus/2(accel)
  Demux/2 -> signalBus/3(gyro)
  Subsystem3/2(Out2) -> Frame Transfer1/1(In1), Add1/2, Subsystem1/2(Inport1)
  Subsystem3/1(accel) -> Frame Transfer/1(In1), Add/2, Subsystem/2(Inport1)
  Bus Selector/3 -> Subsystem3/4(<dw_Body>)  "<dw_Body>"
  flag/1 -> Subsystem3/1(flag)
  Frame Transfer/1(Out1) -> Mux/1
  Frame Transfer1/1(Out1) -> Mux/2

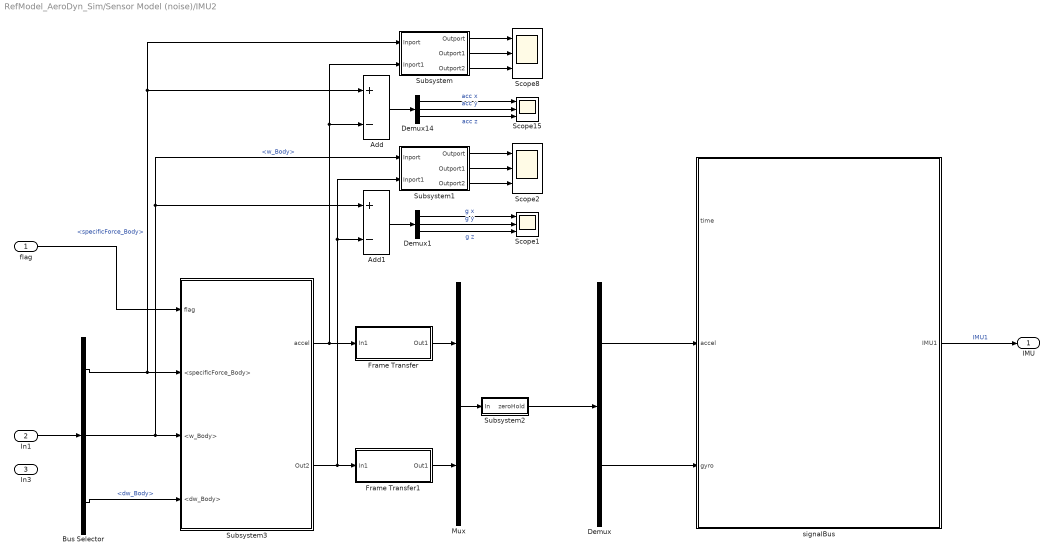
== system RefModel_AeroDyn_Sim/Sensor Model (noise)/IMU2 ==
  flag : Inport
  In1 : Inport  Port=2
  In3 : Inport  Port=3
  Add : Sum  Inputs=+-
  Add1 : Sum  Inputs=+-
  Bus Selector : BusSelector  OutputSignals=specificForce_Body,w_Body,dw_Body
  Demux : Demux  Outputs=2
  Demux1 : Demux  Outputs=3
  Demux14 : Demux  Outputs=3
  Frame Transfer : Subsystem
  Frame Transfer1 : Subsystem
  Mux : Mux  Inputs=2
  Scope{1..2,8,15} (4 alike) : Scope  NumInputPorts=3
  Subsystem : Subsystem
  Subsystem1 : Subsystem
  Subsystem2 : Subsystem  mask{sample_freq=sensorFs.imuUpdateFs}
      mask prompts: sample_freq "采样频率(Hz)"
  Subsystem3 : Subsystem
  signalBus : Subsystem
  IMU : Outport
  wires:
  In1/1 -> Bus Selector/1
  Bus Selector/2 -> Add1/1, Subsystem1/1(Inport), Subsystem3/3(<w_Body>)  "<w_Body>"
  Bus Selector/1 -> Add/1, Subsystem/1(Inport), Subsystem3/2(<specificForce_Body>)  "<specificForce_Body>"
  Add/1 -> Demux14/1
  Demux14/3 -> Scope15/3  "acc z"
  Subsystem/3(Outport2) -> Scope8/3
  Demux14/2 -> Scope15/2  "acc y"
  Demux14/1 -> Scope15/1  "acc x"
  Subsystem/1(Outport) -> Scope8/1
  Subsystem/2(Outport1) -> Scope8/2
  Subsystem1/2(Outport1) -> Scope2/2
  Subsystem1/1(Outport) -> Scope2/1
  Demux1/1 -> Scope1/1  "g x"
  Demux1/2 -> Scope1/2  "g y"
  Subsystem1/3(Outport2) -> Scope2/3
  Demux1/3 -> Scope1/3  "g z"
  Add1/1 -> Demux1/1
  signalBus/1(IMU1) -> IMU/1  "IMU1"
  Mux/1 -> Subsystem2/1(In)
  Subsystem2/1(zeroHold) -> Demux/1
  Demux/1 -> signalBus/2(accel)
  Demux/2 -> signalBus/3(gyro)
  Subsystem3/2(Out2) -> Frame Transfer1/1(In1), Add1/2, Subsystem1/2(Inport1)
  Subsystem3/1(accel) -> Frame Transfer/1(In1), Add/2, Subsystem/2(Inport1)
  Bus Selector/3 -> Subsystem3/4(<dw_Body>)  "<dw_Body>"
  flag/1 -> Subsystem3/1(flag)
  Frame Transfer/1(Out1) -> Mux/1
  Frame Transfer1/1(Out1) -> Mux/2

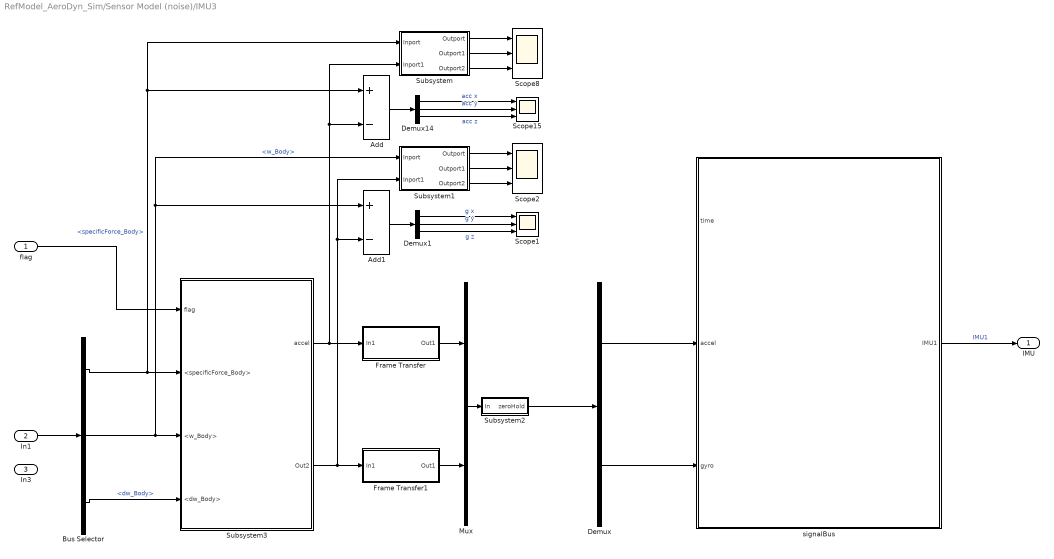
== system RefModel_AeroDyn_Sim/Sensor Model (noise)/IMU3 ==
  flag : Inport
  In1 : Inport  Port=2
  In3 : Inport  Port=3
  Add : Sum  Inputs=+-
  Add1 : Sum  Inputs=+-
  Bus Selector : BusSelector  OutputSignals=specificForce_Body,w_Body,dw_Body
  Demux : Demux  Outputs=2
  Demux1 : Demux  Outputs=3
  Demux14 : Demux  Outputs=3
  Frame Transfer : Subsystem
  Frame Transfer1 : Subsystem
  Mux : Mux  Inputs=2
  Scope{1..2,8,15} (4 alike) : Scope  NumInputPorts=3
  Subsystem : Subsystem
  Subsystem1 : Subsystem
  Subsystem2 : Subsystem  mask{sample_freq=sensorFs.imuUpdateFs}
      mask prompts: sample_freq "采样频率(Hz)"
  Subsystem3 : Subsystem
  signalBus : Subsystem
  IMU : Outport
  wires:
  flag/1 -> Subsystem3/1(flag)
  Bus Selector/3 -> Subsystem3/4(<dw_Body>)  "<dw_Body>"
  Subsystem3/1(accel) -> Subsystem/2(Inport1), Add/2, Frame Transfer/1(In1)
  Subsystem3/2(Out2) -> Subsystem1/2(Inport1), Add1/2, Frame Transfer1/1(In1)
  Demux/2 -> signalBus/3(gyro)
  Demux/1 -> signalBus/2(accel)
  Subsystem2/1(zeroHold) -> Demux/1
  Mux/1 -> Subsystem2/1(In)
  signalBus/1(IMU1) -> IMU/1  "IMU1"
  Add1/1 -> Demux1/1
  Demux1/3 -> Scope1/3  "g z"
  Subsystem1/3(Outport2) -> Scope2/3
  Demux1/2 -> Scope1/2  "g y"
  Demux1/1 -> Scope1/1  "g x"
  Subsystem1/1(Outport) -> Scope2/1
  Subsystem1/2(Outport1) -> Scope2/2
  Subsystem/2(Outport1) -> Scope8/2
  Subsystem/1(Outport) -> Scope8/1
  Demux14/1 -> Scope15/1  "acc x"
  Demux14/2 -> Scope15/2  "acc y"
  Subsystem/3(Outport2) -> Scope8/3
  Demux14/3 -> Scope15/3  "acc z"
  Add/1 -> Demux14/1
  Bus Selector/1 -> Subsystem3/2(<specificForce_Body>), Subsystem/1(Inport), Add/1  "<specificForce_Body>"
  Bus Selector/2 -> Subsystem3/3(<w_Body>), Subsystem1/1(Inport), Add1/1  "<w_Body>"
  In1/1 -> Bus Selector/1
  Frame Transfer/1(Out1) -> Mux/1
  Frame Transfer1/1(Out1) -> Mux/2

== system RefModel_AeroDyn_Sim/Sensor Model (noise)/Mag1 ==
  flag : Inport
  signal : Inport  Port=2
  In3 : Inport  Port=3
  Add : Sum  Inputs=+-
  BodyFrame to MagFrame : Subsystem
  Bus Selector : BusSelector  OutputSignals=mag_Body,magDec_deg
  Demux14 : Demux  Outputs=3
  Gain : Gain
  Scope15 : Scope  NumInputPorts=3
  Scope8 : Scope  NumInputPorts=3
  Subsystem : Subsystem
  Subsystem9 : Subsystem  mask{sample_freq=sensorFs.magUpdateFs}
      mask prompts: sample_freq "采样频率(Hz)"
  add noise : Subsystem
  signalBus : Subsystem
  mag1 : Outport
  wires:
  Bus Selector/1 -> Subsystem/1(Inport), Add/1, add noise/2(signal)  "<mag_Body>"
  signal/1 -> Bus Selector/1
  Demux14/1 -> Scope15/1  "acc x"
  Demux14/2 -> Scope15/2  "acc y"
  Demux14/3 -> Scope15/3  "acc z"
  Add/1 -> Demux14/1
  Subsystem/1(Outport) -> Scope8/1
  Subsystem/2(Outport1) -> Scope8/2
  Subsystem/3(Outport2) -> Scope8/3
  add noise/1(Out1) -> Subsystem/2(Inport1), Add/2, BodyFrame to MagFrame/1(In1)
  BodyFrame to MagFrame/1(Out1) -> Gain/1  "mag1"
  Subsystem9/1(zeroHold) -> signalBus/2(mag)
  signalBus/1(mag1) -> mag1/1  "mag1"
  flag/1 -> add noise/1(noise_flag)
  Gain/1 -> Subsystem9/1(In)

== system RefModel_AeroDyn_Sim/Sensor Model (noise)/Mag2 ==
  flag : Inport
  signal : Inport  Port=2
  In3 : Inport  Port=3
  Add : Sum  Inputs=+-
  BodyFrame to MagFrame : Subsystem
  Bus Selector : BusSelector  OutputSignals=mag_Body,magDec_deg
  Demux14 : Demux  Outputs=3
  Gain : Gain
  Scope15 : Scope  NumInputPorts=3
  Scope8 : Scope  NumInputPorts=3
  Subsystem : Subsystem
  Subsystem9 : Subsystem  mask{sample_freq=sensorFs.magUpdateFs}
      mask prompts: sample_freq "采样频率(Hz)"
  add noise : Subsystem
  signalBus : Subsystem
  mag1 : Outport
  wires:
  flag/1 -> add noise/1(noise_flag)
  signalBus/1(mag1) -> mag1/1  "mag1"
  Subsystem9/1(zeroHold) -> signalBus/2(mag)
  BodyFrame to MagFrame/1(Out1) -> Gain/1  "mag1"
  add noise/1(Out1) -> BodyFrame to MagFrame/1(In1), Add/2, Subsystem/2(Inport1)
  Subsystem/3(Outport2) -> Scope8/3
  Subsystem/2(Outport1) -> Scope8/2
  Subsystem/1(Outport) -> Scope8/1
  Add/1 -> Demux14/1
  Demux14/3 -> Scope15/3  "acc z"
  Demux14/2 -> Scope15/2  "acc y"
  Demux14/1 -> Scope15/1  "acc x"
  signal/1 -> Bus Selector/1
  Bus Selector/1 -> add noise/2(signal), Add/1, Subsystem/1(Inport)  "<mag_Body>"
  Gain/1 -> Subsystem9/1(In)

== system RefModel_AeroDyn_Sim/Sensor Model (noise)/Radar1 ==
  flag : Inport
  In1 : Inport  Port=2
  In3 : Inport  Port=3
  Add : Sum  Inputs=+-
  Bus Selector : BusSelector  OutputSignals=pos_NED
  Gain : Gain  Gain=-1
  Scope8 : Scope  NumInputPorts=2
  Selector : Selector  InputPortWidth=3  IndexOptions=Index vector (dialog)  Indices=3  OutputSizes=1
  Subsystem : Subsystem
  Subsystem3 : Subsystem  mask{sample_freq=sensorFs.radarUpdateFs}
      mask prompts: sample_freq "采样频率(Hz)"
  add noise1 : Subsystem
  radar1 : Subsystem
  range : Outport
  wires:
  Selector/1 -> Gain/1
  Bus Selector/1 -> Selector/1  "<pos_NED>"
  In1/1 -> Bus Selector/1
  add noise1/1(Out1) -> Subsystem3/1(In), Subsystem/2(Inport1), Add/2
  Gain/1 -> add noise1/2(signal), Subsystem/1(Inport), Add/1
  Subsystem/1(Outport) -> Scope8/1
  Add/1 -> Scope8/2
  Subsystem3/1(zeroHold) -> radar1/4(Range)  "radar1"
  radar1/1(radar1) -> range/1  "radar1"
  flag/1 -> add noise1/1(noise_flag)

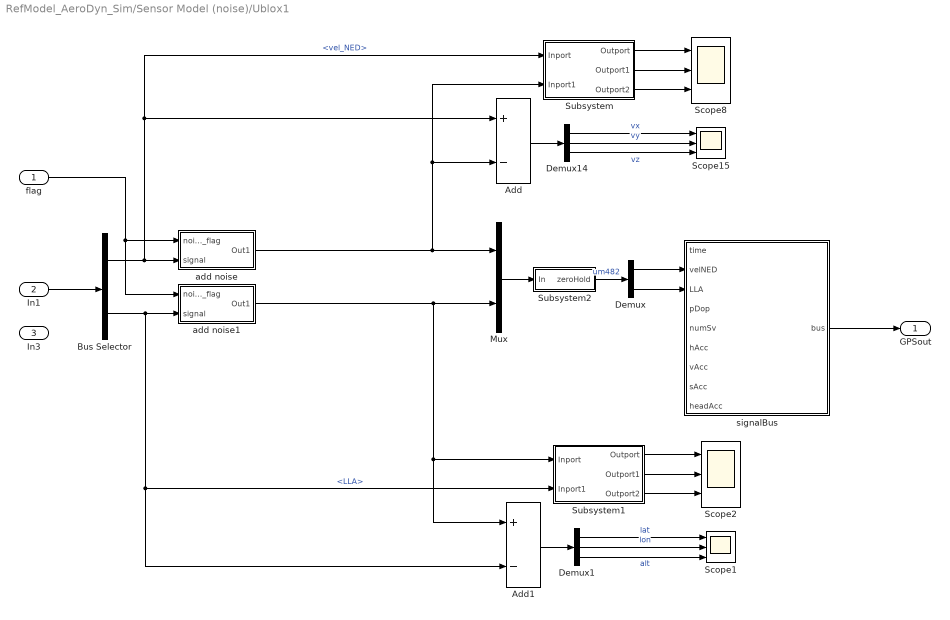
== system RefModel_AeroDyn_Sim/Sensor Model (noise)/Ublox1 ==
  flag : Inport
  In1 : Inport  Port=2
  In3 : Inport  Port=3
  Add : Sum  Inputs=+-
  Add1 : Sum  Inputs=+-
  Bus Selector : BusSelector  OutputSignals=vel_NED,LLA
  Demux : Demux  Outputs=2
  Demux1 : Demux  Outputs=3
  Demux14 : Demux  Outputs=3
  Mux : Mux  Inputs=2
  Scope{1..2,8,15} (4 alike) : Scope  NumInputPorts=3
  Subsystem : Subsystem
  Subsystem1 : Subsystem
  Subsystem2 : Subsystem  mask{sample_freq=sensorFs.gpsUpdateFs}
      mask prompts: sample_freq "采样频率(Hz)"
  add noise : Subsystem
  add noise1 : Subsystem
  signalBus : Subsystem
  GPSout : Outport
  wires:
  In1/1 -> Bus Selector/1
  Bus Selector/2 -> Subsystem1/2(Inport1), Add1/2, add noise1/2(signal)  "<LLA>"
  Bus Selector/1 -> add noise/2(signal), Add/1, Subsystem/1(Inport)  "<vel_NED>"
  add noise/1(Out1) -> Subsystem/2(Inport1), Add/2, Mux/1
  Subsystem/2(Outport1) -> Scope8/2
  Demux14/1 -> Scope15/1  "vx"
  Subsystem/1(Outport) -> Scope8/1
  Subsystem/3(Outport2) -> Scope8/3
  Demux14/2 -> Scope15/2  "vy"
  Add/1 -> Demux14/1
  Demux14/3 -> Scope15/3  "vz"
  Demux1/3 -> Scope1/3  "alt"
  Add1/1 -> Demux1/1
  Demux1/2 -> Scope1/2  "lon"
  Subsystem1/3(Outport2) -> Scope2/3
  Subsystem1/1(Outport) -> Scope2/1
  Demux1/1 -> Scope1/1  "lat"
  Subsystem1/2(Outport1) -> Scope2/2
  add noise1/1(Out1) -> Mux/2, Add1/1, Subsystem1/1(Inport)
  Mux/1 -> Subsystem2/1(In)
  Subsystem2/1(zeroHold) -> Demux/1  "um482"
  Demux/1 -> signalBus/2(velNED)
  Demux/2 -> signalBus/3(LLA)
  signalBus/1(bus) -> GPSout/1
  flag/1 -> add noise/1(noise_flag), add noise1/1(noise_flag)
